simulink subsystem "Derivative"  (R2022b)
settings: Solver=VariableStepAuto  StartTime=0.0  StopTime=10.0  RelTol=1e-3
model mask{Gain=1.0, Init=0, SampleTime=-1, Ts=auto}
  mask prompts: Gain "Gain Value"; Init "Initial Condition"; SampleTime "Simulink:blkprm_prompts:AllBlksSampleTime"
settings Model: Creator=MAAM  LastModifiedBy=MAAM

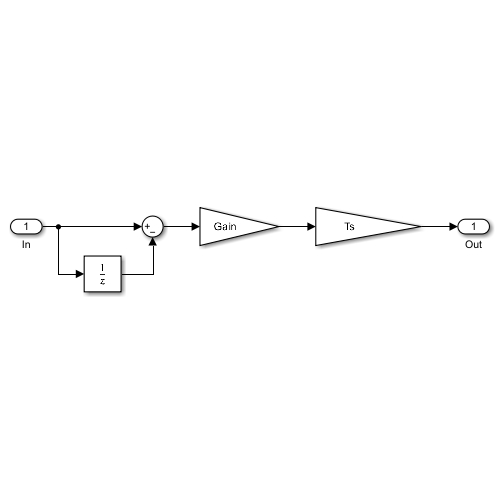
[thumbnail: Simulink's stored preview of the top-level diagram]
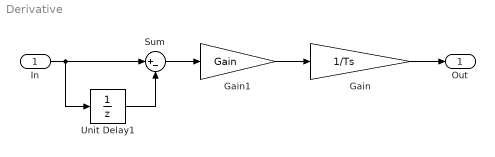
== system Derivative ==
  In : Inport
  Gain : Gain  Gain=1/Ts
  Gain1 : Gain  Gain=Gain
  Sum : Sum  Inputs=|+-
  Unit Delay1 : UnitDelay  SampleTime=-1  HasFrameUpgradeWarning=on
  Out : Outport
  wires:
  Sum/1 -> Gain1/1
  In/1 -> Unit Delay1/1, Sum/1
  Gain1/1 -> Gain/1
  Unit Delay1/1 -> Sum/2
  Gain/1 -> Out/1
